simulink model "VCIMD2_C_R2014a"  (R2014a)
settings: Solver=ode45  StartTime=0.0  StopTime=2.5  RelTol=1e-3
undefined symbols (not defined in the file): Lm, Lr, Rr
libraries: powerlib_meascontrol x16, powerlib x4
settings Model: Creator=Yugal  LastModifiedBy=Yugal
settings DebuggingCC: UnderspecifiedInitializationDetection=Classic
settings SimscapeCC: EditingMode=Restricted

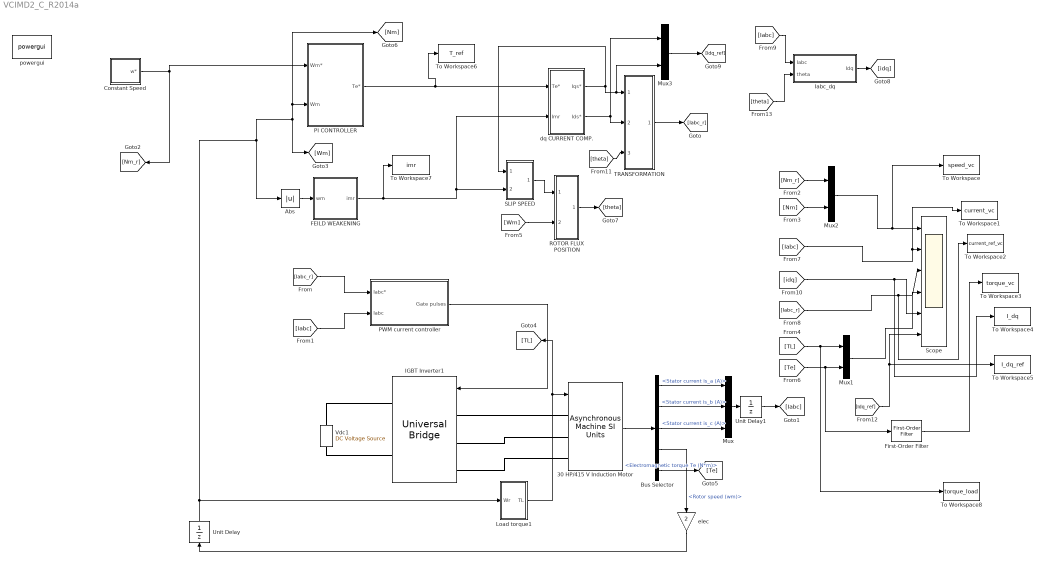
== system VCIMD2_C_R2014a ==
  30 HP/415 V Induction Motor : powerlib/Machines/Asynchronous Machine SI Units  PresetModel=No  MechanicalLoad=Torque Tm  ShowDetailedParameters=on  RotorType=Squirrel-cage  ReferenceFrame=Rotor  Units=SI  MeasurementBus=off  NominalParameters=[30*746 415 50]  Stator=[0.251 0.001397]  Rotor=[Rr 0.001397]  Cage1=[ 0.022 0.226/377]  Cage2=[ 0.022 0.226/377]  Lm=0.0416  Mechanical=[0.305 0 2 ]  PolePairs=2  InitialConditions=[1 0 0 0 0 0 0 0]  SimulateSaturation=off  Saturation=[14.03593122, 27.81365428, 53.79336849, 72.68890987, 97.98006896, 148.6815601, 215.7428561, 302.9841135, 420.4778367 ; 230, 322, 414, 460, 506, 552, 598, 644, 690]  LoadFlowParameters=1492000  TsPowergui=0  TsBlock=-1  IterativeModel=Trapezoidal non iterative  Pmec=0
  Abs : Abs  SaturateOnIntegerOverflow=on
  Bus Selector : BusSelector  OutputSignals=Stator measurements.Stator current is_a (A),Stator measurements.Stator current is_b (A),Stator measurements.Stator current is_c (A),Mechanical.Rotor speed (wm),Mechanical.Electromagnetic torque Te (N*m)
  Constant Speed : Subsystem
  FEILD WEAKENING : MATLAB Function  TreatAsAtomicUnit=on
  First-Order Filter : powerlib_meascontrol/Filters/First-Order Filter  FilterType=Lowpass  Tc=10e-3  Ts=0  Initialize=on  Vac_Init=[0, 0, 60]  Vdc_Init=0  PlotResponse=off  FreqRange="[0,  200,  1]"
  IGBT Inverter1 : powerlib/Power Electronics/Universal Bridge  Arms=3  SnubberResistance=1e5  SnubberCapacitance=inf  Device=MOSFET / Diodes  Ron=1e-3  Lon=0  ForwardVoltages="[  0  0  ]"  ForwardVoltage=0  GTOparameters=[ 10e-6 , 20e-6 ]  IGBTparameters=[ 1e-6 , 2e-6 ]  Measurements=None  Measurements_2=None  converterType=Rectifier
  Iabc_dq : Subsystem
  Load torque1 : Subsystem
  Mux : Mux  Inputs=3
  Mux1 : Mux  Inputs=2
  Mux2 : Mux  Inputs=2
  Mux3 : Mux  Inputs=2
  PI CONTROLLER : Subsystem  mask{Kp=90, Ki=2, Ts=100e-6, Lim=225}
      mask prompts: Ts "Sampling Time Ts (sec)"; Lim "Ref Torque limit(N-m)"
  PWM current controller : Subsystem
  ROTOR FLUX POSITION : Subsystem
  SLIP SPEED : Subsystem
  Scope : Scope  NumInputPorts=6
      settings: TickLabels=on  TimeRange=4  YMin=300~-150~-200~-50~-25~-25  YMax=475~150~200~300~150~175  MaxDataPoints=1000  Decimation=10
  TRANSFORMATION : Subsystem
  To Workspace : ToWorkspace  VariableName=speed_vc  SaveFormat=Structure With Time  SampleTime=100e-6
  To Workspace1 : ToWorkspace  VariableName=current_vc  SaveFormat=Structure With Time  SampleTime=100e-6
  To Workspace2 : ToWorkspace  VariableName=current_ref_vc  SaveFormat=Structure With Time  SampleTime=100e-6
  To Workspace3 : ToWorkspace  VariableName=torque_vc  SaveFormat=Structure With Time  SampleTime=100e-6
  To Workspace4 : ToWorkspace  VariableName=I_dq  SaveFormat=Structure With Time  SampleTime=100e-6
  To Workspace5 : ToWorkspace  VariableName=I_dq_ref  SaveFormat=Structure With Time  SampleTime=100e-6
  To Workspace6 : ToWorkspace  VariableName=T_ref  SaveFormat=Structure With Time  SampleTime=100e-6
  To Workspace7 : ToWorkspace  VariableName=imr  SaveFormat=Structure With Time  SampleTime=100e-6
  To Workspace8 : ToWorkspace  VariableName=torque_load  SaveFormat=Structure With Time  SampleTime=100e-6
  Unit Delay : UnitDelay  SampleTime=100e-6
  Unit Delay1 : UnitDelay  SampleTime=10e-6
  Vdc1 : powerlib/Electrical Sources/DC Voltage Source  Amplitude=560.45  Measurements=None
  dq CURRENT COMP. : Subsystem
  elec : Gain  Gain=2
  powergui : powerlib/powergui  Priority=1  SimulationMode=Discrete  SolverType=Tustin  SampleTime=10e-6  frequency=60  SPID=off  DisableSnubberDevices=off  DisableRonSwitches=off  DisableVfSwitches=off  SwTol=0  Interpol=off  DisplayEquations=off  Ts=0  methode=off  frequencyindice=50  Pbase=100e6  ErrMax=1e-4  Iterations=50  UnitsV=kV  UnitsW=MW  FunctionMessages=off  echomessages=off  HookPort=off  EnableUseOfTLC=off  x0status=blocks  RestoreLinks=warning  ResistiveCurrentMeasurement=off  Frange=[0:2:500]  Ylog=off  Xlog=on  ShowGrid=off  save=off  variable=ZData  structure=current_ref_vc  ZoomFFT=off  StartTime=2  cycles=5  DisplayStyle=4  fundamental=50  FreqAxis=off  MaxFrequency=10000  frequencyindicesteady=1  RmsSteady=1  display=off
  wires:
  PWM current controller/1(Gate pulses) -> IGBT Inverter1/1
  Load torque1/1(TL) -> [TL], 30 HP/415 V Induction Motor/1
  30 HP/415 V Induction Motor/1 -> Bus Selector/1
  Bus Selector/3 -> Mux/3  "<Stator current is_c (A)>"
  Bus Selector/2 -> Mux/2  "<Stator current is_b (A)>"
  Bus Selector/1 -> Mux/1  "<Stator current is_a (A)>"
  [Iabc] -> PWM current controller/2(Iabc)
  [Iabc_r] -> PWM current controller/1(Iabc*)
  Abs/1 -> FEILD WEAKENING/1(wm)
  dq CURRENT COMP./2(Ids*) -> TRANSFORMATION/2(Ids*), Mux3/1
  dq CURRENT COMP./1(Iqs*) -> Mux3/2, TRANSFORMATION/1(Iqs*), SLIP SPEED/1(Iqs*)
  PI CONTROLLER/1(Te*) -> dq CURRENT COMP./1(Te*), To Workspace6/1
  FEILD WEAKENING/1(imr) -> SLIP SPEED/2(Imr*), dq CURRENT COMP./2(Imr), To Workspace7/1
  SLIP SPEED/1(Wsl) -> ROTOR FLUX POSITION/1("Wsl\t")
  [Wm] -> ROTOR FLUX POSITION/2(Wm)
  TRANSFORMATION/1(Iabc*) -> [Iabc_r]
  Bus Selector/5 -> [Te]  "<Electromagnetic torque Te (N*m)>"
  [TL] -> To Workspace8/1, Mux1/1
  Bus Selector/4 -> elec/1  "<Rotor speed (wm)>"
  Mux1/1 -> Scope/4
  [Nm_r] -> Mux2/1
  [Nm] -> Mux2/2
  Mux2/1 -> To Workspace/1, Scope/1
  [Iabc] -> To Workspace1/1, Scope/2
  Constant Speed/1(w*) -> PI CONTROLLER/1(Wm*), [Nm_r]
  [Iabc_r] -> To Workspace2/1, Scope/3
  Mux/1 -> Unit Delay1/1
  Unit Delay1/1 -> [Iabc]
  elec/1 -> Unit Delay/1
  Unit Delay/1 -> Load torque1/1(Wr), [Nm], PI CONTROLLER/2(Wm), [Wm], Abs/1
  ROTOR FLUX POSITION/1(theta) -> [theta]
  [Iabc] -> Iabc_dq/1(Iabc)
  Iabc_dq/1(Idq) -> [idq]
  [idq] -> To Workspace4/1, Scope/5
  [theta] -> TRANSFORMATION/3(theta)
  Mux3/1 -> [Idq_ref]
  [Idq_ref] -> To Workspace5/1, Scope/6
  [theta] -> Iabc_dq/2(theta)
  [Te] -> First-Order Filter/1, Mux1/2
  First-Order Filter/1 -> To Workspace3/1
  connections:
  Vdc1/RConn1 -- IGBT Inverter1/RConn1
  30 HP/415 V Induction Motor/LConn2 -- IGBT Inverter1/LConn2
  Vdc1/LConn1 -- IGBT Inverter1/RConn2
  30 HP/415 V Induction Motor/LConn3 -- IGBT Inverter1/LConn3
  30 HP/415 V Induction Motor/LConn1 -- IGBT Inverter1/LConn1

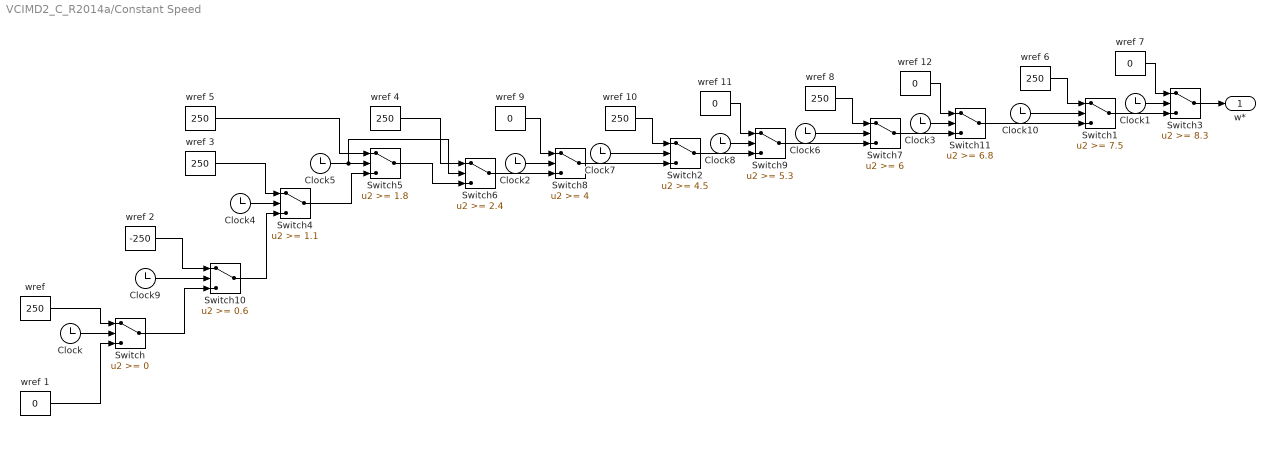
== system VCIMD2_C_R2014a/Constant Speed ==
  Clock{,1..10} (11 alike) : Clock
      settings: Decimation=2
  Switch : Switch  SaturateOnIntegerOverflow=on  InputSameDT=on
  Switch1 : Switch  Threshold=7.5  SaturateOnIntegerOverflow=on  InputSameDT=on
  Switch10 : Switch  Threshold=0.6  SaturateOnIntegerOverflow=on  InputSameDT=on
  Switch11 : Switch  Threshold=6.8  SaturateOnIntegerOverflow=on  InputSameDT=on
  Switch2 : Switch  Threshold=4.5  SaturateOnIntegerOverflow=on  InputSameDT=on
  Switch3 : Switch  Threshold=8.3  SaturateOnIntegerOverflow=on  InputSameDT=on
  Switch4 : Switch  Threshold=1.1  SaturateOnIntegerOverflow=on  InputSameDT=on
  Switch5 : Switch  Threshold=1.8  SaturateOnIntegerOverflow=on  InputSameDT=on
  Switch6 : Switch  Threshold=2.4  SaturateOnIntegerOverflow=on  InputSameDT=on
  Switch7 : Switch  Threshold=6  SaturateOnIntegerOverflow=on  InputSameDT=on
  Switch8 : Switch  Threshold=4  SaturateOnIntegerOverflow=on  InputSameDT=on
  Switch9 : Switch  Threshold=5.3  SaturateOnIntegerOverflow=on  InputSameDT=on
  wref {,3..6,8,10} (7 alike) : Constant  Value=250
  wref {1,7,9,11..12} (5 alike) : Constant  Value=0
  wref 2 : Constant  Value=-250
  w* : Outport
  wires:
  wref 1/1 -> Switch/3
  Clock/1 -> Switch/2
  "wref "/1 -> Switch/1
  Clock4/1 -> Switch4/2
  wref 3/1 -> Switch4/1
  Switch4/1 -> Switch5/3
  Switch5/1 -> Switch6/3
  Clock5/1 -> Switch6/2, Switch5/2
  wref 4/1 -> Switch6/1
  wref 5/1 -> Switch5/1
  Switch10/1 -> Switch4/3
  Switch6/1 -> Switch8/3
  wref 9/1 -> Switch8/1
  Clock2/1 -> Switch8/2
  Switch8/1 -> Switch2/3
  Clock7/1 -> Switch2/2
  wref 10/1 -> Switch2/1
  Switch2/1 -> Switch9/3
  Clock8/1 -> Switch9/2
  wref 11/1 -> Switch9/1
  Switch/1 -> Switch10/3
  Clock9/1 -> Switch10/2
  wref 2/1 -> Switch10/1
  Switch11/1 -> Switch1/3
  Clock10/1 -> Switch1/2
  wref 6/1 -> Switch1/1
  Switch1/1 -> Switch3/3
  Clock1/1 -> Switch3/2
  wref 7/1 -> Switch3/1
  Clock6/1 -> Switch7/2
  wref 8/1 -> Switch7/1
  Switch7/1 -> Switch11/3
  Clock3/1 -> Switch11/2
  wref 12/1 -> Switch11/1
  Switch9/1 -> Switch7/3
  Switch3/1 -> w*/1

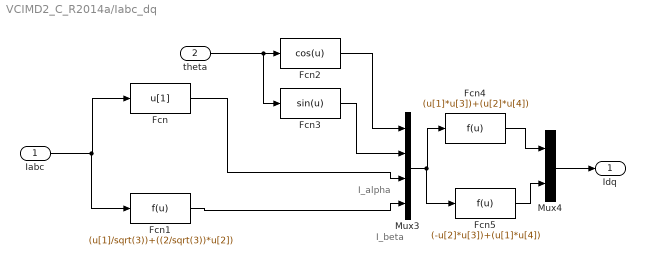
== system VCIMD2_C_R2014a/Iabc_dq ==
  note: I_beta
  note: I_alpha
  Iabc : Inport
  theta : Inport  Port=2
  Fcn : Fcn  Expr=u[1]
  Fcn1 : Fcn  Expr=(u[1]/sqrt(3))+((2/sqrt(3))*u[2])
  Fcn2 : Fcn  Expr=cos(u)
  Fcn3 : Fcn  Expr=sin(u)
  Fcn4 : Fcn  Expr=(u[1]*u[3])+(u[2]*u[4])
  Fcn5 : Fcn  Expr=(-u[2]*u[3])+(u[1]*u[4])
  Mux3 : Mux
  Mux4 : Mux  Inputs=2
  Idq : Outport
  wires:
  Iabc/1 -> Fcn1/1, Fcn/1
  theta/1 -> Fcn3/1, Fcn2/1
  Fcn2/1 -> Mux3/1
  Fcn3/1 -> Mux3/2
  Fcn/1 -> Mux3/3
  Mux3/1 -> Fcn5/1, Fcn4/1
  Fcn4/1 -> Mux4/1
  Fcn5/1 -> Mux4/2
  Mux4/1 -> Idq/1
  Fcn1/1 -> Mux3/4

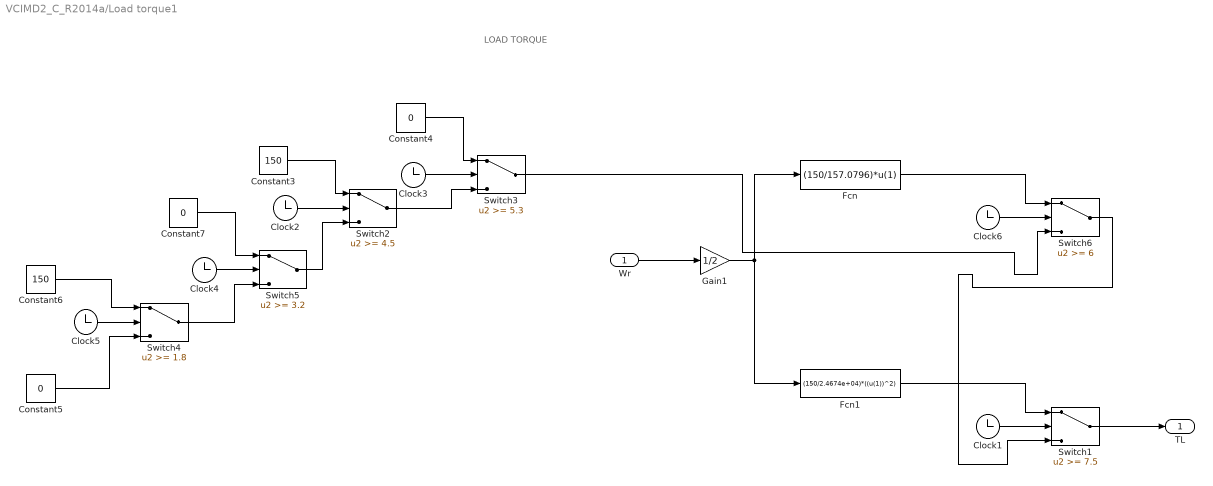
== system VCIMD2_C_R2014a/Load torque1 ==
  note: LOAD TORQUE
  Wr : Inport
  Clock{1..6} (6 alike) : Clock
  Constant3 : Constant  Value=150
  Constant4 : Constant  Value=0
  Constant5 : Constant  Value=0
  Constant6 : Constant  Value=150
  Constant7 : Constant  Value=0
  Fcn : Fcn  Expr=(150/157.0796)*u(1)
  Fcn1 : Fcn  Expr=(150/2.4674e+04)*((u(1))^2)
  Gain1 : Gain  Gain=1/2
  Switch1 : Switch  Threshold=7.5
  Switch2 : Switch  Threshold=4.5
  Switch3 : Switch  Threshold=5.3
  Switch4 : Switch  Threshold=1.8
  Switch5 : Switch  Threshold=3.2
  Switch6 : Switch  Threshold=6
  TL : Outport
  wires:
  Switch5/1 -> Switch2/3
  Clock2/1 -> Switch2/2
  Switch2/1 -> Switch3/3
  Clock3/1 -> Switch3/2
  Constant3/1 -> Switch2/1
  Constant4/1 -> Switch3/1
  Wr/1 -> Gain1/1
  Gain1/1 -> Fcn/1, Fcn1/1
  Constant5/1 -> Switch4/3
  Constant6/1 -> Switch4/1
  Switch4/1 -> Switch5/3
  Clock4/1 -> Switch5/2
  Constant7/1 -> Switch5/1
  Clock5/1 -> Switch4/2
  Clock6/1 -> Switch6/2
  Fcn/1 -> Switch6/1
  Switch3/1 -> Switch6/3
  Clock1/1 -> Switch1/2
  Fcn1/1 -> Switch1/1
  Switch6/1 -> Switch1/3
  Switch1/1 -> TL/1

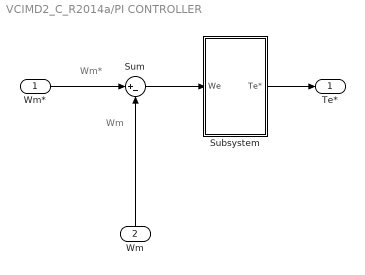
== system VCIMD2_C_R2014a/PI CONTROLLER ==
  note: Wm*
  note: Wm
  Wm* : Inport
  Wm : Inport  Port=2
  Subsystem : Subsystem
  Sum : Sum  Inputs=|+-
  Te* : Outport
  wires:
  Wm*/1 -> Sum/1
  Subsystem/1(Te*) -> Te*/1
  Sum/1 -> Subsystem/1(We)
  Wm/1 -> Sum/2

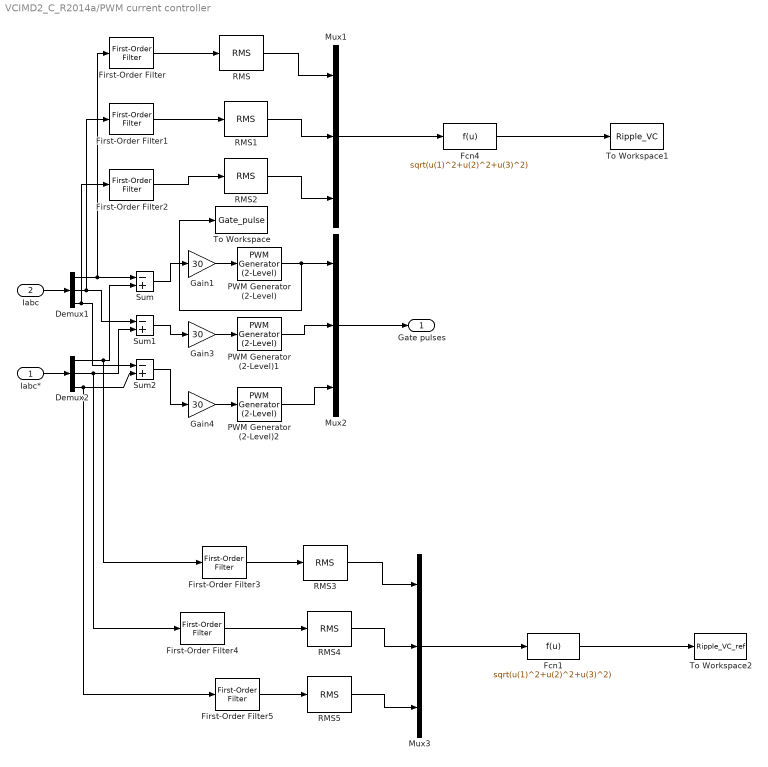
== system VCIMD2_C_R2014a/PWM current controller ==
  Iabc* : Inport
  Iabc : Inport  Port=2
  Demux1 : Demux  Outputs=3
  Demux2 : Demux  Outputs=3
  Fcn1 : Fcn  Expr=sqrt(u(1)^2+u(2)^2+u(3)^2)
  Fcn4 : Fcn  Expr=sqrt(u(1)^2+u(2)^2+u(3)^2)
  First-Order Filter : powerlib_meascontrol/Filters/First-Order Filter  FilterType=Highpass  Tc=0.5e-3  Ts=0  Initialize=on  Vac_Init=[0, 0, 60]  Vdc_Init=0  PlotResponse=off  FreqRange="[0,  200,  1]"
  First-Order Filter1 : powerlib_meascontrol/Filters/First-Order Filter  FilterType=Highpass  Tc=0.5e-3  Ts=0  Initialize=on  Vac_Init=[0, 0, 60]  Vdc_Init=0  PlotResponse=off  FreqRange="[0,  200,  1]"
  First-Order Filter2 : powerlib_meascontrol/Filters/First-Order Filter  FilterType=Highpass  Tc=0.5e-3  Ts=0  Initialize=on  Vac_Init=[0, 0, 60]  Vdc_Init=0  PlotResponse=off  FreqRange="[0,  200,  1]"
  First-Order Filter3 : powerlib_meascontrol/Filters/First-Order Filter  FilterType=Highpass  Tc=0.5e-3  Ts=0  Initialize=on  Vac_Init=[0, 0, 50]  Vdc_Init=0  PlotResponse=off  FreqRange="[0,  200,  1]"
  First-Order Filter4 : powerlib_meascontrol/Filters/First-Order Filter  FilterType=Highpass  Tc=0.5e-3  Ts=0  Initialize=on  Vac_Init=[0, 0, 50]  Vdc_Init=0  PlotResponse=off  FreqRange="[0,  200,  1]"
  First-Order Filter5 : powerlib_meascontrol/Filters/First-Order Filter  FilterType=Highpass  Tc=0.5e-3  Ts=0  Initialize=on  Vac_Init=[0, 0, 50]  Vdc_Init=0  PlotResponse=off  FreqRange="[0,  200,  1]"
  Gain1 : Gain  Gain=30  SaturateOnIntegerOverflow=on  OutDataTypeStr=Inherit: Same as input  ParamDataTypeStr=Inherit: Same as input
  Gain3 : Gain  Gain=30  SaturateOnIntegerOverflow=on  OutDataTypeStr=Inherit: Same as input  ParamDataTypeStr=Inherit: Same as input
  Gain4 : Gain  Gain=30  SaturateOnIntegerOverflow=on  OutDataTypeStr=Inherit: Same as input  ParamDataTypeStr=Inherit: Same as input
  Mux1 : Mux  Inputs=3
  Mux2 : Mux  Inputs=3
  Mux3 : Mux  Inputs=3
  PWM Generator (2-Level) : powerlib_meascontrol/Pulse & Signal Generators/PWM Generator (2-Level)  ModulatorType=Single-phase half-bridge (2 pulses)  ModulatorMode=Unsynchronized  nF=27  Fc=10000  ModulatingSignals=off  m=0.8  Freq=60  Phase=0  Ts=10e-6
  PWM Generator (2-Level)1 : powerlib_meascontrol/Pulse & Signal Generators/PWM Generator (2-Level)  ModulatorType=Single-phase half-bridge (2 pulses)  ModulatorMode=Unsynchronized  nF=27  Fc=10000  ModulatingSignals=off  m=0.8  Freq=60  Phase=0  Ts=5e-6
  PWM Generator (2-Level)2 : powerlib_meascontrol/Pulse & Signal Generators/PWM Generator (2-Level)  ModulatorType=Single-phase half-bridge (2 pulses)  ModulatorMode=Unsynchronized  nF=27  Fc=10000  ModulatingSignals=off  m=0.8  Freq=60  Phase=0  Ts=5e-6
  RMS : powerlib_meascontrol/Measurements/RMS  TrueRMS=on  Freq=60  RMSInit=120  Ts=0
  RMS1 : powerlib_meascontrol/Measurements/RMS  TrueRMS=on  Freq=60  RMSInit=120  Ts=0
  RMS2 : powerlib_meascontrol/Measurements/RMS  TrueRMS=on  Freq=60  RMSInit=120  Ts=0
  RMS3 : powerlib_meascontrol/Measurements/RMS  TrueRMS=off  Freq=50  RMSInit=0  Ts=0
  RMS4 : powerlib_meascontrol/Measurements/RMS  TrueRMS=off  Freq=50  RMSInit=0  Ts=0
  RMS5 : powerlib_meascontrol/Measurements/RMS  TrueRMS=off  Freq=50  RMSInit=0  Ts=0
  Sum : Sum  Inputs=-+  SaturateOnIntegerOverflow=on  InputSameDT=on  OutDataTypeStr=Inherit: Same as first input
  Sum1 : Sum  Inputs=-+  SaturateOnIntegerOverflow=on  InputSameDT=on  OutDataTypeStr=Inherit: Same as first input
  Sum2 : Sum  Inputs=-+  SaturateOnIntegerOverflow=on  InputSameDT=on  OutDataTypeStr=Inherit: Same as first input
  To Workspace : ToWorkspace  VariableName=Gate_pulse  SaveFormat=Structure With Time  SampleTime=100e-6
  To Workspace1 : ToWorkspace  VariableName=Ripple_VC  SaveFormat=Structure With Time  SampleTime=100e-6
  To Workspace2 : ToWorkspace  VariableName=Ripple_VC_ref  SaveFormat=Structure With Time  SampleTime=100e-6
  Gate pulses : Outport
  wires:
  PWM Generator (2-Level)/1 -> To Workspace/1, Mux2/1
  PWM Generator (2-Level)1/1 -> Mux2/2
  PWM Generator (2-Level)2/1 -> Mux2/3
  Gain3/1 -> PWM Generator (2-Level)1/1
  Gain4/1 -> PWM Generator (2-Level)2/1
  Mux2/1 -> Gate pulses/1
  Gain1/1 -> PWM Generator (2-Level)/1
  Demux1/1 -> First-Order Filter/1, Sum/1
  Iabc/1 -> Demux1/1
  Demux1/3 -> First-Order Filter2/1, Sum2/1
  Iabc*/1 -> Demux2/1
  Sum/1 -> Gain1/1
  Sum1/1 -> Gain3/1
  Sum2/1 -> Gain4/1
  Demux1/2 -> First-Order Filter1/1, Sum1/1
  First-Order Filter/1 -> RMS/1
  First-Order Filter1/1 -> RMS1/1
  First-Order Filter2/1 -> RMS2/1
  RMS2/1 -> Mux1/3
  RMS1/1 -> Mux1/2
  RMS/1 -> Mux1/1
  Mux1/1 -> Fcn4/1
  Fcn4/1 -> To Workspace1/1
  Demux2/1 -> First-Order Filter3/1, Sum/2
  Demux2/2 -> First-Order Filter4/1, Sum1/2
  Demux2/3 -> First-Order Filter5/1, Sum2/2
  RMS5/1 -> Mux3/3
  RMS4/1 -> Mux3/2
  RMS3/1 -> Mux3/1
  Mux3/1 -> Fcn1/1
  Fcn1/1 -> To Workspace2/1
  First-Order Filter3/1 -> RMS3/1
  First-Order Filter4/1 -> RMS4/1
  First-Order Filter5/1 -> RMS5/1

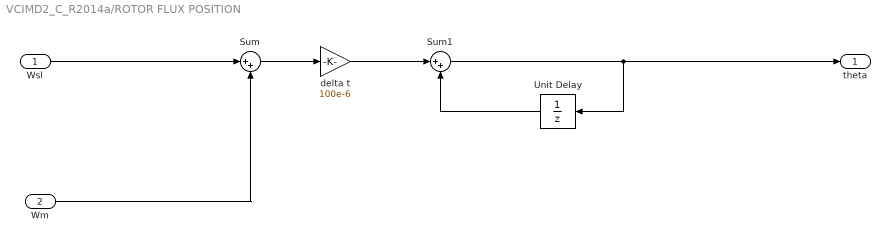
== system VCIMD2_C_R2014a/ROTOR FLUX POSITION ==
  "Wsl\t" : Inport
  Wm : Inport  Port=2
  Sum : Sum  Inputs=|++
  Sum1 : Sum  Inputs=|++
  Unit Delay : UnitDelay  SampleTime=100e-6
  delta t : Gain  Gain=100e-6
  theta : Outport
  wires:
  delta t/1 -> Sum1/1
  Sum1/1 -> theta/1, Unit Delay/1
  Sum/1 -> delta t/1
  Unit Delay/1 -> Sum1/2
  Wm/1 -> Sum/2
  "Wsl\t"/1 -> Sum/1

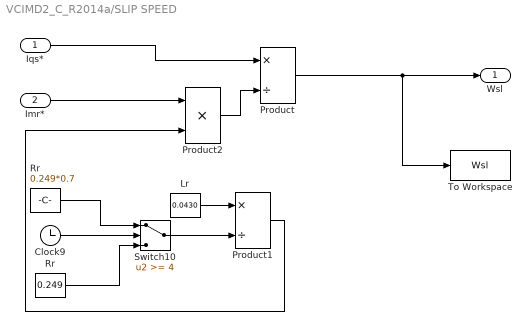
== system VCIMD2_C_R2014a/SLIP SPEED ==
  Iqs* : Inport
  Imr* : Inport  Port=2
  Clock9 : Clock
      settings: Decimation=2
  Lr : Constant  Value=0.0430
  Product : Product  Inputs=*/
  Product1 : Product  Inputs=*/
  Product2 : Product  Inputs=**
  Rr : Constant  Value=0.249*0.7
  "Rr " : Constant  Value=0.249
  Switch10 : Switch  Threshold=4  SaturateOnIntegerOverflow=on  InputSameDT=on
  To Workspace : ToWorkspace  VariableName=Wsl  SaveFormat=Structure With Time  SampleTime=100e-6
  Wsl : Outport
  wires:
  Iqs*/1 -> Product/1
  Product2/1 -> Product/2
  Imr*/1 -> Product2/1
  Clock9/1 -> Switch10/2
  "Rr "/1 -> Switch10/3
  Rr/1 -> Switch10/1
  Switch10/1 -> Product1/2
  Lr/1 -> Product1/1
  Product1/1 -> Product2/2
  Product/1 -> To Workspace/1, Wsl/1

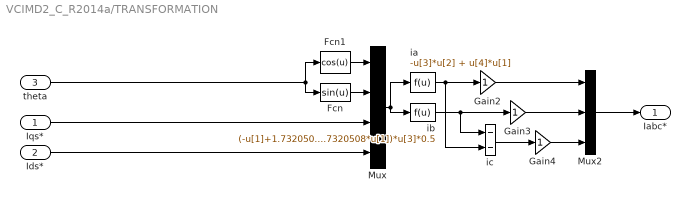
== system VCIMD2_C_R2014a/TRANSFORMATION ==
  Iqs* : Inport
  Ids* : Inport  Port=2
  theta : Inport  Port=3
  Fcn : Fcn  Expr=sin(u)
  Fcn1 : Fcn  Expr=cos(u)
  Gain2 : Gain  SaturateOnIntegerOverflow=on  OutDataTypeStr=Inherit: Same as input  ParamDataTypeStr=Inherit: Same as input
  Gain3 : Gain  SaturateOnIntegerOverflow=on  OutDataTypeStr=Inherit: Same as input  ParamDataTypeStr=Inherit: Same as input
  Gain4 : Gain  SaturateOnIntegerOverflow=on  OutDataTypeStr=Inherit: Same as input  ParamDataTypeStr=Inherit: Same as input
  Mux : Mux
  Mux2 : Mux  Inputs=3
  ia : Fcn  Expr=-u[3]*u[2] + u[4]*u[1]
  ib : Fcn  Expr=(-u[1]+1.7320508*u[2])*u[4]*0.5+(u[2]+1.7320508*u[1])*u[3]*0.5
  ic : Sum  Inputs=--  SaturateOnIntegerOverflow=on  InputSameDT=on  OutDataTypeStr=Inherit: Same as first input
  Iabc* : Outport
  wires:
  Fcn/1 -> Mux/2
  theta/1 -> Fcn/1, Fcn1/1
  Mux2/1 -> Iabc*/1
  Gain3/1 -> Mux2/2
  Fcn1/1 -> Mux/1
  ic/1 -> Gain4/1
  ib/1 -> Gain3/1, ic/1
  Mux/1 -> ib/1, ia/1
  ia/1 -> Gain2/1, ic/2
  Iqs*/1 -> Mux/3
  Ids*/1 -> Mux/4
  Gain2/1 -> Mux2/1
  Gain4/1 -> Mux2/3

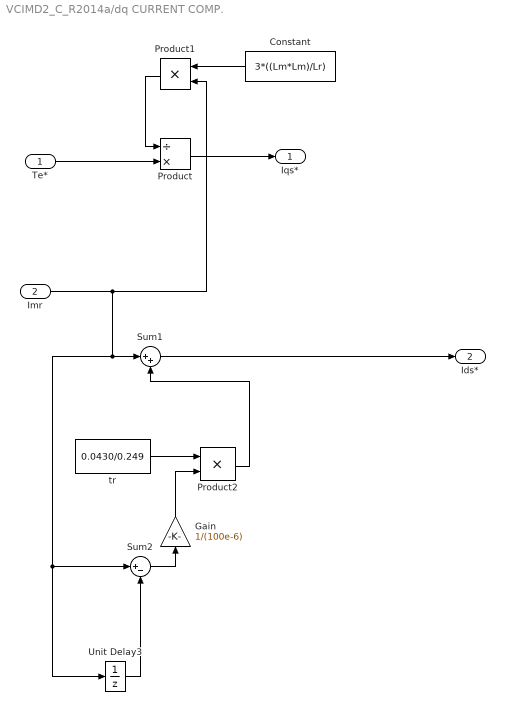
== system VCIMD2_C_R2014a/dq CURRENT COMP. ==
  Te* : Inport
  Imr : Inport  Port=2
  Constant : Constant  Value=3*((Lm*Lm)/Lr)
  Gain : Gain  Gain=1/(100e-6)
  Product : Product  Inputs=/*
  Product1 : Product
  Product2 : Product  SaturateOnIntegerOverflow=on  InputSameDT=on  OutDataTypeStr=Inherit: Same as first input
  Sum1 : Sum  Inputs=|++
  Sum2 : Sum  Inputs=|+-
  Unit Delay3 : UnitDelay  SampleTime=100e-6
  tr : Constant  Value=0.0430/0.249
  Iqs* : Outport
  Ids* : Outport  Port=2
  wires:
  Product1/1 -> Product/1
  Constant/1 -> Product1/1
  Te*/1 -> Product/2
  Product/1 -> Iqs*/1
  Imr/1 -> Sum2/1, Unit Delay3/1, Sum1/1, Product1/2
  tr/1 -> Product2/1
  Product2/1 -> Sum1/2
  Sum1/1 -> Ids*/1
  Unit Delay3/1 -> Sum2/2
  Sum2/1 -> Gain/1
  Gain/1 -> Product2/2

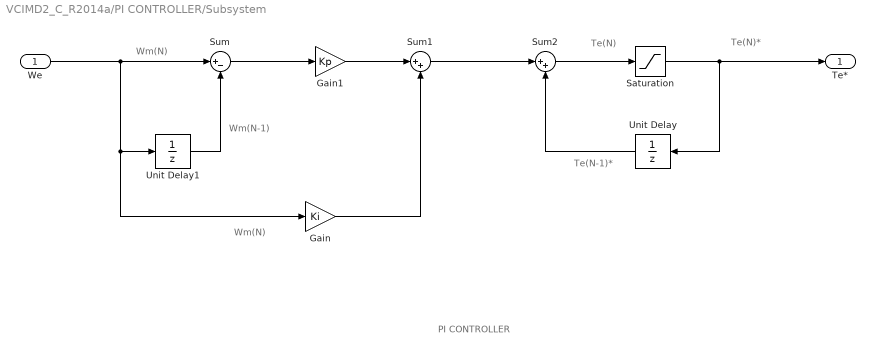
== system VCIMD2_C_R2014a/PI CONTROLLER/Subsystem ==
  note: PI CONTROLLER
  note: Wm(N)
  note: Wm(N-1)
  note: Wm(N)
  note: Te(N)
  note: Te(N)*
  note: Te(N-1)*
  We : Inport
  Gain : Gain  Gain=Ki
  Gain1 : Gain  Gain=Kp
  Saturation : Saturate  UpperLimit=Lim  LowerLimit=-Lim
  Sum : Sum  Inputs=|+-
  Sum1 : Sum  Inputs=|++
  Sum2 : Sum  Inputs=|++
  Unit Delay : UnitDelay  SampleTime=Ts
  Unit Delay1 : UnitDelay  SampleTime=Ts
  Te* : Outport
  wires:
  Sum1/1 -> Sum2/1
  Sum2/1 -> Saturation/1
  Saturation/1 -> Unit Delay/1, Te*/1
  Sum/1 -> Gain1/1
  Gain1/1 -> Sum1/1
  Unit Delay1/1 -> Sum/2
  We/1 -> Sum/1, Unit Delay1/1, Gain/1
  Gain/1 -> Sum1/2
  Unit Delay/1 -> Sum2/2

== matlab function VCIMD2_C_R2014a/FEILD WEAKENING ==
  data: wm input; imr output
function imr = fcn(wm)
%#codegen
if wm<2*pi*50
   imr=21.6;
else
    imr=2*pi*50*21.6/wm;
end
